simulink model "adaptable2D"  (Simulink 6.0)
settings: Solver=ode45  StartTime=0.0  StopTime=inf  RelTol=1e-3
libraries: simulink x2, spelookup x1
settings Model: Creator=beryilma  LastModifiedBy=rlandy
settings DataIOCC: SaveOutput=off  SaveTime=off  SignalLoggingName=sigsOut
settings OptimizationCC: BooleanDataType=off
settings DebuggingCC: CheckExecutionContextPreStartOutputMsg=on  CheckExecutionContextRuntimeOutputMsg=on  SolverPrmCheckMsg=none
settings HardwareCC: TargetUnknown=on
settings ModelReferenceCC: UpdateModelReferenceTargets=IfOutOfDate
settings GRTTargetCC: LifeSpan=inf
settings SFSimCC: SFSimApplyToAllLibs=on  SFSimBuildMode=Incremental

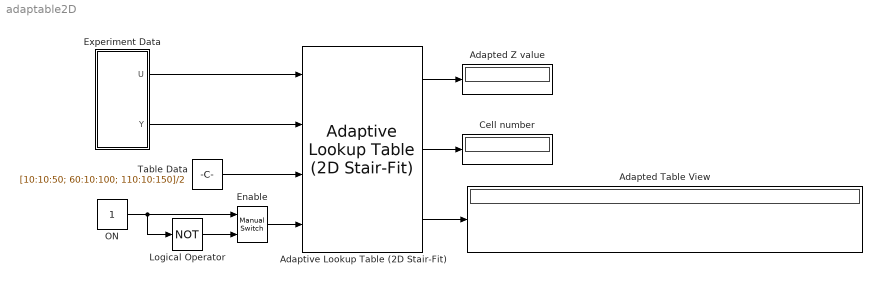
== system adaptable2D ==
  Adapted Table View : Display
  Adapted Z value : Display
  Adaptive Lookup Table (2D Stair-Fit) : spelookup/Adaptive Lookup Table (2D Stair-Fit)  Bp_Row=[1 2 3 4]  Bp_Column=[0 1 2 3 4 5]  Tb_Input=on  Tb_Data=[10:10:50; 60:10:100; 110:10:150]  Tb_NumData=reshape(1:15,3,5)  Ad_Method=Sample mean (with forgetting)  Ad_Factor=0.96  Tb_Output=on  Ad_Enable=on  Ad_Lock=off  Ad_Range=Ignore
  Cell number : Display
  Enable : simulink/Signal Routing/Manual Switch  sw=1  action=0
  Experiment Data : Subsystem  EnableExecutionContextPropagation=on
  Logical Operator : Logic  Operator=NOT
  ON : Constant
  Table Data : Constant  Value=[10:10:50; 60:10:100; 110:10:150]/2
  wires:
  ON/1 -> Logical Operator/1, Enable/1
  Logical Operator/1 -> Enable/2
  Adaptive Lookup Table (2D Stair-Fit)/1 -> Adapted Z value/1
  Adaptive Lookup Table (2D Stair-Fit)/2 -> Cell number/1
  Experiment Data/1(U) -> Adaptive Lookup Table (2D Stair-Fit)/1
  Experiment Data/2(Y) -> Adaptive Lookup Table (2D Stair-Fit)/2
  Adaptive Lookup Table (2D Stair-Fit)/3 -> Adapted Table View/1
  Table Data/1 -> Adaptive Lookup Table (2D Stair-Fit)/3
  Enable/1 -> Adaptive Lookup Table (2D Stair-Fit)/4

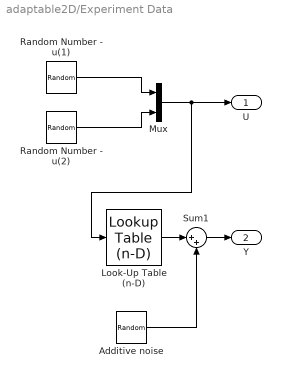
== system adaptable2D/Experiment Data ==
  Additive noise : UniformRandomNumber  Maximum=+1  Seed=1  SampleTime=0
  Look-Up Table (n-D) : simulink/Lookup Tables/Lookup Table (n-D)  numDimsPopupSelect=2  bp1=[1.5 2.5 3.5]  bp2=[0.5 1.5 2.5 3.5 4.5]  bp3=[1:3]  bp4=[1:3]  bpcell={ [1:3], [1:3] }  explicitNumDims=2  searchMode=Binary Search  cacheBpFlag=off  vectorInputFlag=on  tableData=[10:10:50; 60:10:100; 110:10:150]  interpMethod=Linear  extrapMethod=Linear  rangeErrorMode=None
  Mux : Mux  Inputs=2
  Random Number - u(1) : UniformRandomNumber  Minimum=0  Maximum=5  Seed=3  SampleTime=0
  Random Number - u(2) : UniformRandomNumber  Maximum=6  Seed=7  SampleTime=0
  Sum1 : Sum  Inputs=|++  SaturateOnIntegerOverflow=on  InputSameDT=on
  U : Outport
  Y : Outport  Port=2
  wires:
  Additive noise/1 -> Sum1/2
  Random Number - u(1)/1 -> Mux/1
  Random Number - u(2)/1 -> Mux/2
  Mux/1 -> U/1, Look-Up Table (n-D)/1
  Sum1/1 -> Y/1
  Look-Up Table (n-D)/1 -> Sum1/1
